simulink model "batt_electrics_RUL_SOC"  (R2022a)
settings: Solver=FixedStepAuto  StartTime=0.0  StopTime=1800*100  FixedStep=1e-1  RelTol=1e-3
undefined symbols (not defined in the file or in its folder): DiscIntNeverNeededParam
libraries: ee_lib x16, nesl_utility x6, fl_lib x4, simulink x1, dspstat3 x1
(part 1 of 3)
settings Model: Creator=OADEBAJO  LastModifiedBy=OADEBAJO

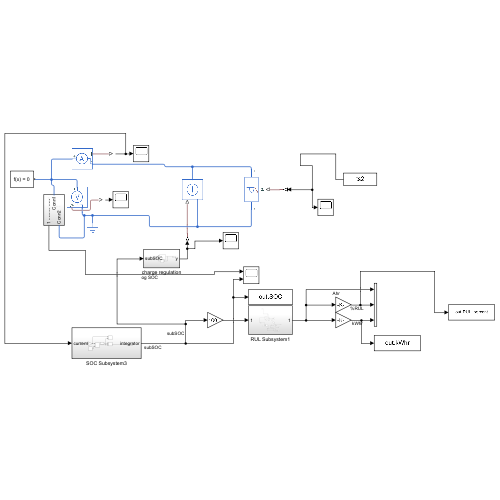
[thumbnail: Simulink's stored preview of the top-level diagram]
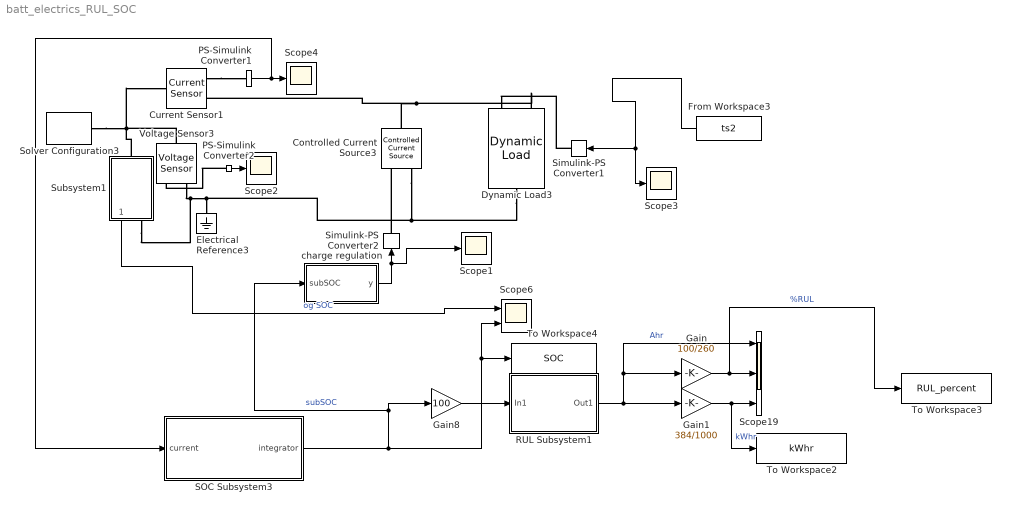
== system batt_electrics_RUL_SOC ==
  Controlled Current Source3 : fl_lib/Electrical/Electrical Sources/Controlled Current Source
      settings: SourceProductBaseCode=PW,SS,VE
  Current Sensor1 : fl_lib/Electrical/Electrical Sensors/Current Sensor
      settings: SourceProductBaseCode=PW,SS,VE
  Dynamic Load3 : ee_lib/Passive/Dynamic Load  load_type=ee.enum.dc_ac.dc  min_supply_voltage=20 V  pow_min=1e-3 W  G_reverse=1e-6 S  deltaV=1e-3 V  f0=60 Hz  Vrms_min=200 V  Pmin=1e-3 W  enable_fault=simscape.enum.onoff.off  fault_action=simscape.enum.assert.action.none  t_fault=1 s  open_conductance=1e-4 S
      settings: SourceProductBaseCode=PS  InternalSimscapePortConfiguration="{\"Bottom\":[],\"Left\":[{\"id\":\"p\",\"label\":\"+\",\"type\":\"foundation.electrical.electrical\"}],\"Right\":[{\"id\":\"n\",\"label\":\"-\",\"type\":\"foundation.electrical.electrical\"}],\"Top\":[{\"id\":\"P\",\"label\":\"P\",\"type\":\"input\"}]}"
  Electrical Reference3 : fl_lib/Electrical/Electrical Elements/Electrical Reference
      settings: SourceProductBaseCode=PW,SS,VE
  From Workspace3 : FromWorkspace  VariableName=ts2
  Gain : Gain  Gain=100/260
  Gain1 : Gain  Gain=384/1000
  Gain8 : Gain  Gain=100
  PS-Simulink Converter1 : nesl_utility/PS-Simulink Converter  PhysicalDomain=network_engine_domain  SubClassName=ps_output  LeftPortType=input  RightPortType=output  PseudoPeriodic=off  Frequencies=[]  VectorFormat=inherit  Unit=inherit  AffineConversion=off
      settings: SourceProductBaseCode=SS,PW,VE
  PS-Simulink Converter2 : nesl_utility/PS-Simulink Converter  PhysicalDomain=network_engine_domain  SubClassName=ps_output  LeftPortType=input  RightPortType=output  PseudoPeriodic=off  Frequencies=[]  VectorFormat=inherit  Unit=inherit  AffineConversion=off
      settings: SourceProductBaseCode=SS,PW,VE
  RUL Subsystem1 : Subsystem
  SOC Subsystem3 : Subsystem
  Scope{1..4} (4 alike) : Scope
  Scope19 : Scope  NumInputPorts=3
  Scope6 : Scope  NumInputPorts=2
  Simulink-PS Converter1 : nesl_utility/Simulink-PS Converter  PhysicalDomain=network_engine_domain  SubClassName=ps_input  LeftPortType=input  RightPortType=output  PseudoPeriodic=off  Frequencies=[]  NoiseDistribution=none  NoiseParameters=[]  Unit=1  AffineConversion=off  FilteringAndDerivatives=provide  SimscapeFilterOrder=1  InputFilterTimeConstant=0.001  UdotUserProvided=0
      settings: SourceProductBaseCode=SS,PW,VE
  Simulink-PS Converter2 : nesl_utility/Simulink-PS Converter  PhysicalDomain=network_engine_domain  SubClassName=ps_input  LeftPortType=input  RightPortType=output  PseudoPeriodic=off  Frequencies=[]  NoiseDistribution=none  NoiseParameters=[]  Unit=1  AffineConversion=off  FilteringAndDerivatives=provide  SimscapeFilterOrder=1  InputFilterTimeConstant=0.001  UdotUserProvided=0
      settings: SourceProductBaseCode=SS,PW,VE
  Solver Configuration3 : nesl_utility/Solver Configuration  PhysicalDomain=network_engine_domain  SubClassName=solver  LeftPortType=input  RightPortType=generic  Tones=[]  Harmonics=[]  SimulateNoise=off  Profile=off  UseLocalSampling=off  EnableSwitchedLinearOptims=on  FrequencyDomain=off  UseCCode=off  RelTol=0.001  AbsTol=0.001  MinStep=1e-09  ToWorkspace=off  RevertToSquareIcSolve=off  NumHomotopyIterations=100  PhasorMode=off  PhasorModeNumHarmonics=1  IndexReductionMethod=DerivativeReplacement  DoDC=off  ResidualTolerance=1e-09  UseLocalSolver=off  LocalSolverChoice=NE_BACKWARD_EULER_ADVANCER  LocalSolverSampleTime=0.001  DoFixedCost=off  MaxNonlinIter=3  MaxModeIter=2  ComputeImpulses=off  ImpulseIterations=2  LinearAlgebra=auto  LinearAlgebraNumThread=0  EquationFormulation=NE_TIME_EF  DelaysMemoryBudget=1024  AutomaticFiltering=on  FilteringTimeConstant=0.001  PartitionStorageMethod=AS_NEEDED  PartitionMemoryBudget=1024  PartitionMethod=ROBUST
      settings: SourceProductBaseCode=SS,PW,VE
  Subsystem1 : Subsystem
  To Workspace2 : ToWorkspace  VariableName=kWhr  SaveFormat=Timeseries  SampleTime=-1
  To Workspace3 : ToWorkspace  VariableName=RUL_percent  SaveFormat=Timeseries  SampleTime=-1
  To Workspace4 : ToWorkspace  VariableName=SOC  SaveFormat=Timeseries  SampleTime=-1
  Voltage Sensor3 : fl_lib/Electrical/Electrical Sensors/Voltage Sensor
      settings: SourceProductBaseCode=PW,SS,VE
  charge regulation : Subsystem
  wires:
  From Workspace3/1 -> Scope3/1, Simulink-PS Converter1/1
  Gain/1 -> To Workspace3/1, Scope19/2  "%RUL"
  SOC Subsystem3/1(integrator) -> Gain8/1, charge regulation/1(subSOC), To Workspace4/1, Scope6/2  "subSOC"
  Gain8/1 -> RUL Subsystem1/1(In1)
  Gain1/1 -> To Workspace2/1, Scope19/3  "kWhr"
  PS-Simulink Converter2/1 -> Scope2/1
  RUL Subsystem1/1(Out1) -> Scope19/1, Gain/1, Gain1/1  "Ahr"
  Subsystem1/1(Out1) -> Scope6/1  "og SOC"
  PS-Simulink Converter1/1 -> Scope4/1, SOC Subsystem3/1(current)
  charge regulation/1(y) -> Scope1/1, Simulink-PS Converter2/1
  connections:
  Voltage Sensor3/RConn2 -- Subsystem1/RConn1 -- Electrical Reference3/LConn1 -- Dynamic Load3/RConn1 -- Controlled Current Source3/RConn2
  Subsystem1/LConn1 -- Solver Configuration3/RConn1 -- Current Sensor1/LConn1 -- Voltage Sensor3/LConn1
  Dynamic Load3/LConn1 -- Controlled Current Source3/LConn1 -- Current Sensor1/RConn2
  Simulink-PS Converter2/RConn1 -- Controlled Current Source3/RConn1
  Current Sensor1/RConn1 -- PS-Simulink Converter1/LConn1
  Simulink-PS Converter1/RConn1 -- Dynamic Load3/LConn2
  PS-Simulink Converter2/LConn1 -- Voltage Sensor3/RConn1

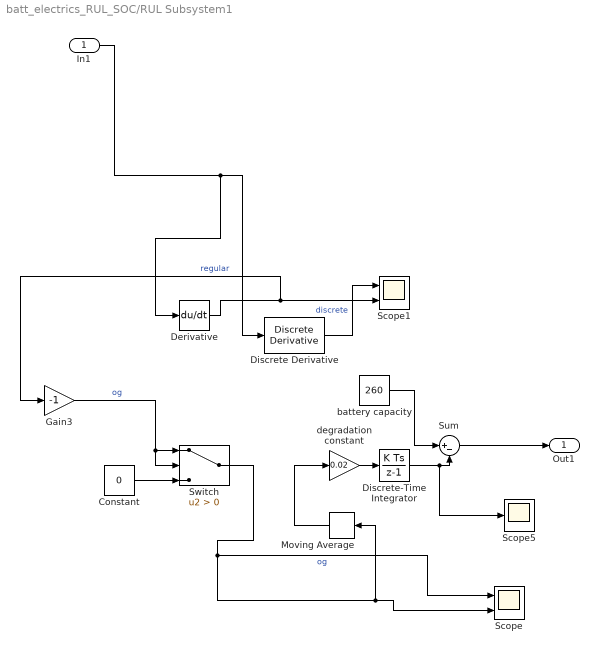
== system batt_electrics_RUL_SOC/RUL Subsystem1 ==
  In1 : Inport
  Constant : Constant  Value=0
  Derivative : Derivative  CoefficientInTFapproximation=1000
  Discrete Derivative : simulink/Discrete/Discrete Derivative  gainval=1.0  ICPrevScaledInput=0.0  OutMin=[]  OutMax=[]  OutDataType=fixdt(1, 16)  OutScaling=2^-10  DoSatur=off
  Discrete-Time Integrator : DiscreteIntegrator  SampleTime=-1  ICPrevOutput=DiscIntNeverNeededParam  ICPrevScaledInput=DiscIntNeverNeededParam
  Gain3 : Gain  Gain=-1
  Moving Average : dspstat3/Moving Average  Method=Sliding window  ForgettingFactorPort=off  SpecifyWindowLength=on  WindowLength=4  ForgettingFactor=0.9  SimulateUsing=Code generation
  Scope : Scope  NumInputPorts=2
  Scope1 : Scope  NumInputPorts=2
  Scope5 : Scope
  Sum : Sum  Inputs=|+-
  Switch : Switch  Criteria=u2 > Threshold  ZeroCross=off  SaturateOnIntegerOverflow=off  InputSameDT=off
  battery capacity : Constant  Value=260
  degradation constant : Gain  Gain=0.02
  Out1 : Outport
  wires:
  Gain3/1 -> Switch/2, Switch/1  "og"
  Constant/1 -> Switch/3
  Derivative/1 -> Gain3/1, Scope1/2  "regular"
  Discrete-Time Integrator/1 -> Scope5/1, Sum/2
  degradation constant/1 -> Discrete-Time Integrator/1
  Discrete Derivative/1 -> Scope1/1  "discrete"
  battery capacity/1 -> Sum/1
  Switch/1 -> Moving Average/1, Scope/2, Scope/1  "og"
  Sum/1 -> Out1/1
  In1/1 -> Derivative/1, Discrete Derivative/1
  Moving Average/1 -> degradation constant/1

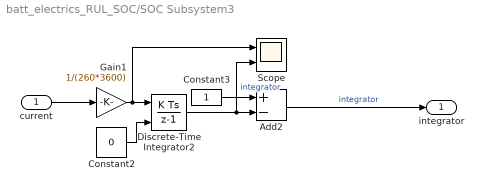
== system batt_electrics_RUL_SOC/SOC Subsystem3 ==
  current : Inport
  Add2 : Sum  Inputs=+-
  Constant2 : Constant  Value=0
  Constant3 : Constant
  Discrete-Time Integrator2 : DiscreteIntegrator  InitialConditionSource=external  SampleTime=-1  ICPrevOutput=DiscIntNeverNeededParam  ICPrevScaledInput=DiscIntNeverNeededParam
  Gain1 : Gain  Gain=1/(260*3600)
  Scope : Scope  NumInputPorts=2
  integrator : Outport
  wires:
  Constant2/1 -> Discrete-Time Integrator2/2
  Constant3/1 -> Add2/1
  current/1 -> Gain1/1
  Gain1/1 -> Scope/1, Discrete-Time Integrator2/1
  Discrete-Time Integrator2/1 -> Scope/2, Add2/2  "integrator"
  Add2/1 -> integrator/1  "integrator"
